simulink model "discretefilter_test_cocoSim_pp"  (Simulink 8.4)
settings: Solver=ode45  StartTime=0.0  StopTime=10.0  RelTol=1e-3
settings Model: Creator=arnaud  LastModifiedBy=arnaud
settings DataIOCC: SaveFormat=Structure  SignalLoggingSaveFormat=Dataset
settings OptimizationCC: ExpressionDepthLimit=128
settings DebuggingCC: UnderspecifiedInitializationDetection=Simplified  MergeDetectMultiDrivingBlocksExec=error  FcnCallInpInsideContextMsg=EnableAllAsError  StateNameClashWarn=none
settings GRTTargetCC: CombineOutputUpdateFcns=on  GRTInterface=off

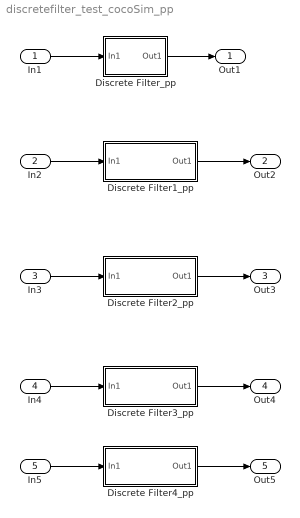
== system discretefilter_test_cocoSim_pp ==
  In1 : Inport
  In2 : Inport  Port=2
  In3 : Inport  Port=3  PortDimensions=3
  In4 : Inport  Port=4  PortDimensions=[2 3]
  In5 : Inport  Port=5  PortDimensions=[1 3]
  Discrete Filter1_pp : Subsystem
  Discrete Filter2_pp : Subsystem
  Discrete Filter3_pp : Subsystem
  Discrete Filter4_pp : Subsystem
  Discrete Filter_pp : Subsystem
  Out1 : Outport
  Out2 : Outport  Port=2
  Out3 : Outport  Port=3
  Out4 : Outport  Port=4
  Out5 : Outport  Port=5
  wires:
  In1/1 -> Discrete Filter_pp/1(In1)
  Discrete Filter_pp/1(Out1) -> Out1/1
  In2/1 -> Discrete Filter1_pp/1(In1)
  Discrete Filter1_pp/1(Out1) -> Out2/1
  In3/1 -> Discrete Filter2_pp/1(In1)
  Discrete Filter2_pp/1(Out1) -> Out3/1
  In4/1 -> Discrete Filter3_pp/1(In1)
  Discrete Filter3_pp/1(Out1) -> Out4/1
  In5/1 -> Discrete Filter4_pp/1(In1)
  Discrete Filter4_pp/1(Out1) -> Out5/1

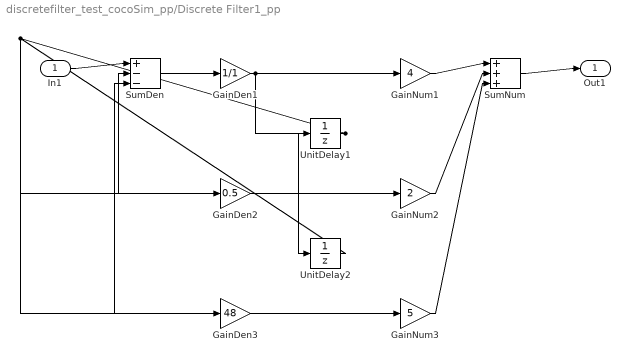
== system discretefilter_test_cocoSim_pp/Discrete Filter1_pp ==
  In1 : Inport
  GainDen1 : Gain  Gain=1/1  SaturateOnIntegerOverflow=on  OutDataTypeStr=Inherit: Same as input  ParamDataTypeStr=Inherit: Same as input
  GainDen2 : Gain  Gain=0.5  SaturateOnIntegerOverflow=on  OutDataTypeStr=Inherit: Same as input  ParamDataTypeStr=Inherit: Same as input
  GainDen3 : Gain  Gain=48  SaturateOnIntegerOverflow=on  OutDataTypeStr=Inherit: Same as input  ParamDataTypeStr=Inherit: Same as input
  GainNum1 : Gain  Gain=4  SaturateOnIntegerOverflow=on  OutDataTypeStr=Inherit: Same as input  ParamDataTypeStr=Inherit: Same as input
  GainNum2 : Gain  Gain=2  SaturateOnIntegerOverflow=on  OutDataTypeStr=Inherit: Same as input  ParamDataTypeStr=Inherit: Same as input
  GainNum3 : Gain  Gain=5  SaturateOnIntegerOverflow=on  OutDataTypeStr=Inherit: Same as input  ParamDataTypeStr=Inherit: Same as input
  SumDen : Sum  Inputs=+--  SaturateOnIntegerOverflow=on  InputSameDT=on  OutDataTypeStr=Inherit: Same as first input
  SumNum : Sum  Inputs=+++  SaturateOnIntegerOverflow=on  InputSameDT=on  OutDataTypeStr=Inherit: Same as first input
  UnitDelay1 : UnitDelay  InitialCondition=1
  UnitDelay2 : UnitDelay  InitialCondition=0.9
  Out1 : Outport
  wires:
  In1/1 -> SumDen/1
  SumNum/1 -> Out1/1
  SumDen/1 -> GainDen1/1
  GainDen2/1 -> SumDen/2
  GainDen3/1 -> SumDen/3
  GainDen1/1 -> GainNum1/1, UnitDelay1/1
  GainNum1/1 -> SumNum/1
  GainNum2/1 -> SumNum/2
  GainNum3/1 -> SumNum/3
  UnitDelay1/1 -> GainDen2/1, GainNum2/1, UnitDelay2/1
  UnitDelay2/1 -> GainDen3/1, GainNum3/1

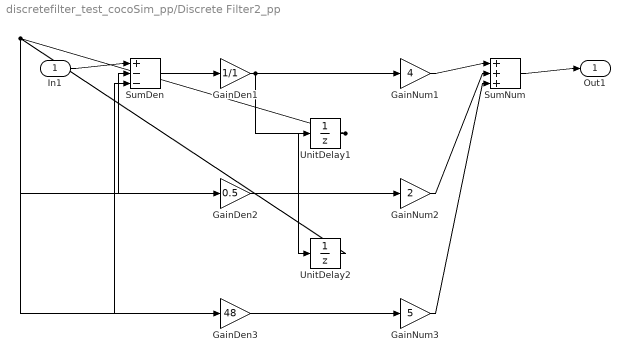
== system discretefilter_test_cocoSim_pp/Discrete Filter2_pp ==
  In1 : Inport
  GainDen1 : Gain  Gain=1/1  SaturateOnIntegerOverflow=on  OutDataTypeStr=Inherit: Same as input  ParamDataTypeStr=Inherit: Same as input
  GainDen2 : Gain  Gain=0.5  SaturateOnIntegerOverflow=on  OutDataTypeStr=Inherit: Same as input  ParamDataTypeStr=Inherit: Same as input
  GainDen3 : Gain  Gain=48  SaturateOnIntegerOverflow=on  OutDataTypeStr=Inherit: Same as input  ParamDataTypeStr=Inherit: Same as input
  GainNum1 : Gain  Gain=4  SaturateOnIntegerOverflow=on  OutDataTypeStr=Inherit: Same as input  ParamDataTypeStr=Inherit: Same as input
  GainNum2 : Gain  Gain=2  SaturateOnIntegerOverflow=on  OutDataTypeStr=Inherit: Same as input  ParamDataTypeStr=Inherit: Same as input
  GainNum3 : Gain  Gain=5  SaturateOnIntegerOverflow=on  OutDataTypeStr=Inherit: Same as input  ParamDataTypeStr=Inherit: Same as input
  SumDen : Sum  Inputs=+--  SaturateOnIntegerOverflow=on  InputSameDT=on  OutDataTypeStr=Inherit: Same as first input
  SumNum : Sum  Inputs=+++  SaturateOnIntegerOverflow=on  InputSameDT=on  OutDataTypeStr=Inherit: Same as first input
  UnitDelay1 : UnitDelay  InitialCondition=1
  UnitDelay2 : UnitDelay  InitialCondition=0.9
  Out1 : Outport
  wires:
  In1/1 -> SumDen/1
  SumNum/1 -> Out1/1
  SumDen/1 -> GainDen1/1
  GainDen2/1 -> SumDen/2
  GainDen3/1 -> SumDen/3
  GainDen1/1 -> GainNum1/1, UnitDelay1/1
  GainNum1/1 -> SumNum/1
  GainNum2/1 -> SumNum/2
  GainNum3/1 -> SumNum/3
  UnitDelay1/1 -> GainDen2/1, GainNum2/1, UnitDelay2/1
  UnitDelay2/1 -> GainDen3/1, GainNum3/1

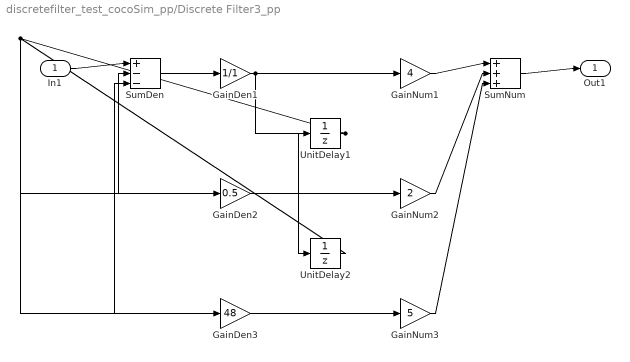
== system discretefilter_test_cocoSim_pp/Discrete Filter3_pp ==
  In1 : Inport
  GainDen1 : Gain  Gain=1/1  SaturateOnIntegerOverflow=on  OutDataTypeStr=Inherit: Same as input  ParamDataTypeStr=Inherit: Same as input
  GainDen2 : Gain  Gain=0.5  SaturateOnIntegerOverflow=on  OutDataTypeStr=Inherit: Same as input  ParamDataTypeStr=Inherit: Same as input
  GainDen3 : Gain  Gain=48  SaturateOnIntegerOverflow=on  OutDataTypeStr=Inherit: Same as input  ParamDataTypeStr=Inherit: Same as input
  GainNum1 : Gain  Gain=4  SaturateOnIntegerOverflow=on  OutDataTypeStr=Inherit: Same as input  ParamDataTypeStr=Inherit: Same as input
  GainNum2 : Gain  Gain=2  SaturateOnIntegerOverflow=on  OutDataTypeStr=Inherit: Same as input  ParamDataTypeStr=Inherit: Same as input
  GainNum3 : Gain  Gain=5  SaturateOnIntegerOverflow=on  OutDataTypeStr=Inherit: Same as input  ParamDataTypeStr=Inherit: Same as input
  SumDen : Sum  Inputs=+--  SaturateOnIntegerOverflow=on  InputSameDT=on  OutDataTypeStr=Inherit: Same as first input
  SumNum : Sum  Inputs=+++  SaturateOnIntegerOverflow=on  InputSameDT=on  OutDataTypeStr=Inherit: Same as first input
  UnitDelay1 : UnitDelay  InitialCondition=1
  UnitDelay2 : UnitDelay  InitialCondition=0.9
  Out1 : Outport
  wires:
  In1/1 -> SumDen/1
  SumNum/1 -> Out1/1
  SumDen/1 -> GainDen1/1
  GainDen2/1 -> SumDen/2
  GainDen3/1 -> SumDen/3
  GainDen1/1 -> GainNum1/1, UnitDelay1/1
  GainNum1/1 -> SumNum/1
  GainNum2/1 -> SumNum/2
  GainNum3/1 -> SumNum/3
  UnitDelay1/1 -> GainDen2/1, GainNum2/1, UnitDelay2/1
  UnitDelay2/1 -> GainDen3/1, GainNum3/1

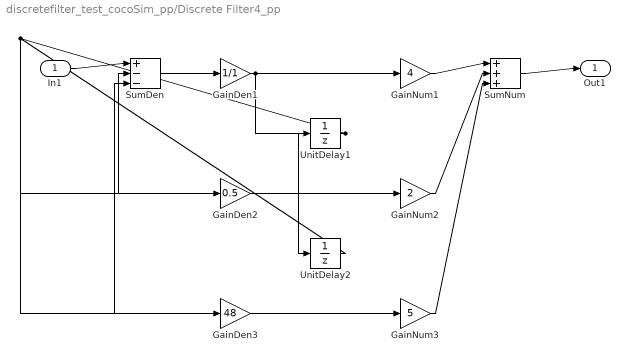
== system discretefilter_test_cocoSim_pp/Discrete Filter4_pp ==
  In1 : Inport
  GainDen1 : Gain  Gain=1/1  SaturateOnIntegerOverflow=on  OutDataTypeStr=Inherit: Same as input  ParamDataTypeStr=Inherit: Same as input
  GainDen2 : Gain  Gain=0.5  SaturateOnIntegerOverflow=on  OutDataTypeStr=Inherit: Same as input  ParamDataTypeStr=Inherit: Same as input
  GainDen3 : Gain  Gain=48  SaturateOnIntegerOverflow=on  OutDataTypeStr=Inherit: Same as input  ParamDataTypeStr=Inherit: Same as input
  GainNum1 : Gain  Gain=4  SaturateOnIntegerOverflow=on  OutDataTypeStr=Inherit: Same as input  ParamDataTypeStr=Inherit: Same as input
  GainNum2 : Gain  Gain=2  SaturateOnIntegerOverflow=on  OutDataTypeStr=Inherit: Same as input  ParamDataTypeStr=Inherit: Same as input
  GainNum3 : Gain  Gain=5  SaturateOnIntegerOverflow=on  OutDataTypeStr=Inherit: Same as input  ParamDataTypeStr=Inherit: Same as input
  SumDen : Sum  Inputs=+--  SaturateOnIntegerOverflow=on  InputSameDT=on  OutDataTypeStr=Inherit: Same as first input
  SumNum : Sum  Inputs=+++  SaturateOnIntegerOverflow=on  InputSameDT=on  OutDataTypeStr=Inherit: Same as first input
  UnitDelay1 : UnitDelay  InitialCondition=1
  UnitDelay2 : UnitDelay  InitialCondition=0.9
  Out1 : Outport
  wires:
  In1/1 -> SumDen/1
  SumNum/1 -> Out1/1
  SumDen/1 -> GainDen1/1
  GainDen2/1 -> SumDen/2
  GainDen3/1 -> SumDen/3
  GainDen1/1 -> GainNum1/1, UnitDelay1/1
  GainNum1/1 -> SumNum/1
  GainNum2/1 -> SumNum/2
  GainNum3/1 -> SumNum/3
  UnitDelay1/1 -> GainDen2/1, GainNum2/1, UnitDelay2/1
  UnitDelay2/1 -> GainDen3/1, GainNum3/1

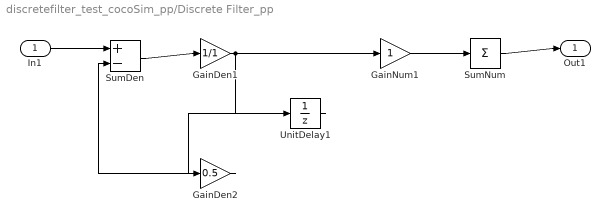
== system discretefilter_test_cocoSim_pp/Discrete Filter_pp ==
  In1 : Inport
  GainDen1 : Gain  Gain=1/1  SaturateOnIntegerOverflow=on  OutDataTypeStr=Inherit: Same as input  ParamDataTypeStr=Inherit: Same as input
  GainDen2 : Gain  Gain=0.5  SaturateOnIntegerOverflow=on  OutDataTypeStr=Inherit: Same as input  ParamDataTypeStr=Inherit: Same as input
  GainNum1 : Gain  SaturateOnIntegerOverflow=on  OutDataTypeStr=Inherit: Same as input  ParamDataTypeStr=Inherit: Same as input
  SumDen : Sum  Inputs=+-  SaturateOnIntegerOverflow=on  InputSameDT=on  OutDataTypeStr=Inherit: Same as first input
  SumNum : Sum  Inputs=+  SaturateOnIntegerOverflow=on  InputSameDT=on  OutDataTypeStr=Inherit: Same as first input
  UnitDelay1 : UnitDelay
  Out1 : Outport
  wires:
  In1/1 -> SumDen/1
  SumNum/1 -> Out1/1
  SumDen/1 -> GainDen1/1
  GainDen2/1 -> SumDen/2
  GainDen1/1 -> GainNum1/1, UnitDelay1/1
  GainNum1/1 -> SumNum/1
  UnitDelay1/1 -> GainDen2/1
